simulink model "LQR"  (R2025b)
settings: Solver=VariableStepAuto  StartTime=0.0  StopTime=50.0  RelTol=1e-3
undefined symbols (not defined in the file): A, B, K_LQR_i, K_LQR_x, n, q1_ref_lqr
settings Model: Creator=salvo  LastModifiedBy=salvo

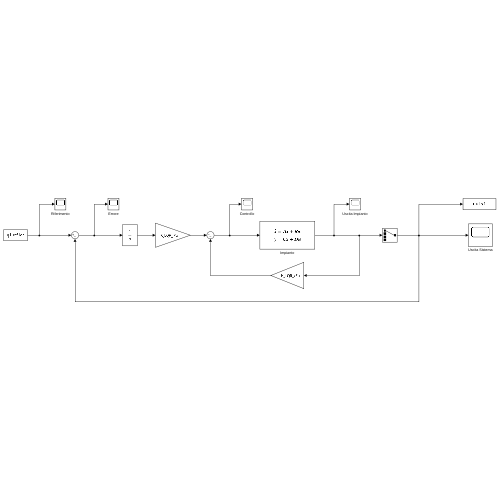
[thumbnail: Simulink's stored preview of the top-level diagram]
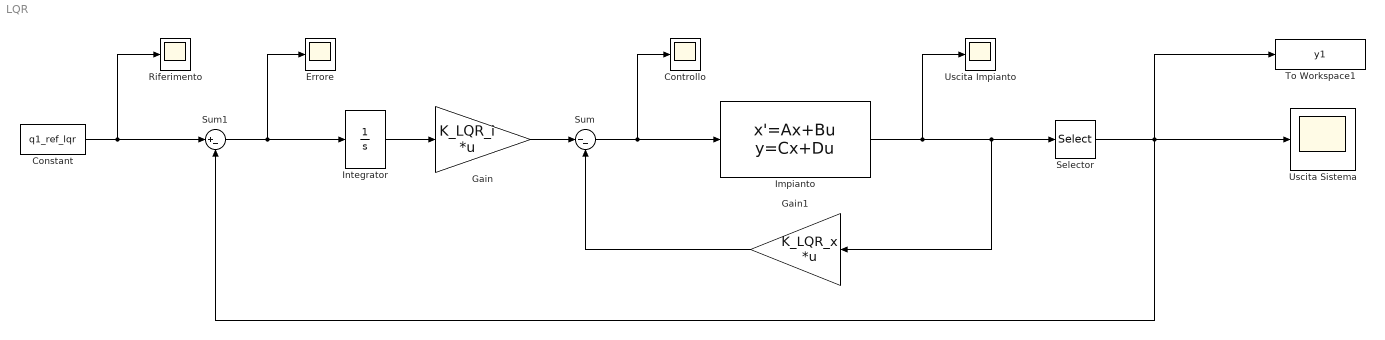
== system LQR ==
  Constant : Constant  Value=q1_ref_lqr
  Controllo : Scope
      settings: ActiveDisplayYMinimum=-50.581356163614664  ActiveDisplayYMaximum=104.42462703199348  DataLoggingVariableName=ScopeData3
  Errore : Scope
      settings: ActiveDisplayYMinimum=0.49728785195365022  ActiveDisplayYMaximum=0.50107619249184232  DataLoggingVariableName=ScopeData2
  Gain : Gain  Gain=K_LQR_i  Multiplication=Matrix(K*u)
  Gain1 : Gain  Gain=K_LQR_x  Multiplication=Matrix(K*u)
  Impianto : StateSpace  A=A  B=B  C=eye(n)  D=zeros(4,2)  InitialCondition=0
  Integrator : Integrator
  Riferimento : Scope
      settings: ActiveDisplayYMinimum=0.4  ActiveDisplayYMaximum=0.6
  Selector : Selector  InputPortWidth=4  IndexOptions=Index vector (dialog)  Indices=[1]  OutputSizes=1
  Sum : Sum  Inputs=|--
  Sum1 : Sum  Inputs=|+-
  To Workspace1 : ToWorkspace  VariableName=y1  SaveFormat=Timeseries  SampleTime=-1
  Uscita Impianto : Scope
      settings: ActiveDisplayYMinimum=-0.52106685941930564  ActiveDisplayYMaximum=4.0853708494874965  DataLoggingVariableName=ScopeData4
  Uscita Sistema : Scope
      settings: ActiveDisplayYMinimum=0.48718369361404734  ActiveDisplayYMaximum=0.50492808194517724
  wires:
  Sum/1 -> Impianto/1, Controllo/1
  Gain1/1 -> Sum/2
  Impianto/1 -> Uscita Impianto/1, Gain1/1, Selector/1
  Selector/1 -> Uscita Sistema/1, To Workspace1/1, Sum1/2
  Constant/1 -> Riferimento/1, Sum1/1
  Gain/1 -> Sum/1
  Integrator/1 -> Gain/1
  Sum1/1 -> Integrator/1, Errore/1
